simulink model "TP1EJ3_2"  (R2024b)
settings: Solver=VariableStepAuto  StartTime=0.0  StopTime=10.0  FixedStep=0.  RelTol=1e-3
values from neighbouring files (symbols this model uses):
  F = zeros(4,1)    [TP1_Entregable.m]
  Ks = 1.2    [TP1_Entregable.m]
  mur = mus(j)    [TP1_Entregable.m]
  n0 = 0    [TP1_Entregable.m]
  p0 = 0    [TP1_Entregable.m]
  Q = zeros(4,1)    [TP1_Entregable.m]
  s0 = 0    [TP1_Entregable.m]
  s_in = 25    [TP1_Entregable.m]
  v0 = 10    [TP1_Entregable.m]
  x0 = 15    [TP1_Entregable.m]
  xi_in = [0,0; s_in,0; 0,n_in; 0,0]    [TP1_Entregable.m]
undefined symbols (not defined in the file or in its folder): sr
settings Model: Creator=tomii  LastModifiedBy=tomi

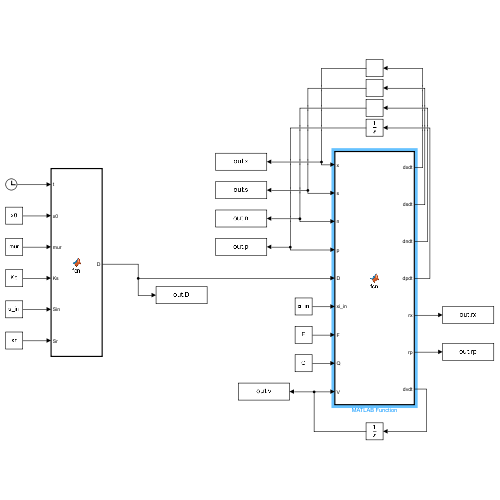
[thumbnail: Simulink's stored preview of the top-level diagram]
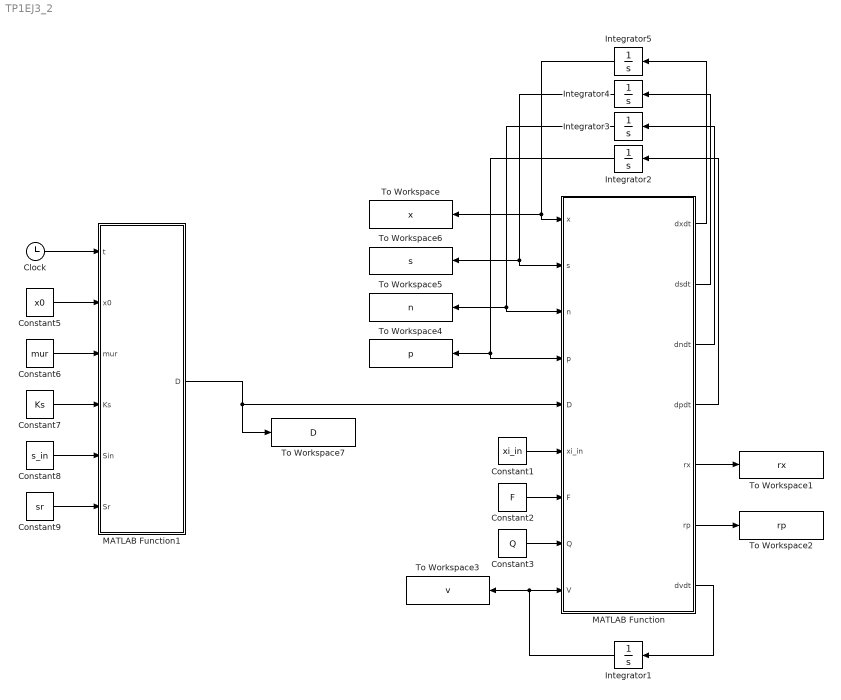
== system TP1EJ3_2 ==
  Clock : Clock
  Constant1 : Constant  Value=xi_in
  Constant2 : Constant  Value=F
  Constant3 : Constant  Value=Q
  Constant5 : Constant  Value=x0
  Constant6 : Constant  Value=mur
  Constant7 : Constant  Value=Ks
  Constant8 : Constant  Value=s_in
  Constant9 : Constant  Value=sr
  Integrator1 : Integrator  InitialCondition=v0
  Integrator2 : Integrator  InitialCondition=p0
  Integrator3 : Integrator  InitialCondition=n0
  Integrator4 : Integrator  InitialCondition=s0
  Integrator5 : Integrator  InitialCondition=x0
  MATLAB Function : MATLAB Function  TreatAsAtomicUnit=on
  MATLAB Function1 : MATLAB Function  TreatAsAtomicUnit=on
  To Workspace : ToWorkspace  VariableName=x  SaveFormat=Timeseries  SampleTime=-1
  To Workspace1 : ToWorkspace  VariableName=rx  SaveFormat=Timeseries  SampleTime=-1
  To Workspace2 : ToWorkspace  VariableName=rp  SaveFormat=Timeseries  SampleTime=-1
  To Workspace3 : ToWorkspace  VariableName=v  SaveFormat=Timeseries  SampleTime=-1
  To Workspace4 : ToWorkspace  VariableName=p  SaveFormat=Timeseries  SampleTime=-1
  To Workspace5 : ToWorkspace  VariableName=n  SaveFormat=Timeseries  SampleTime=-1
  To Workspace6 : ToWorkspace  VariableName=s  SaveFormat=Timeseries  SampleTime=-1
  To Workspace7 : ToWorkspace  VariableName=D  SaveFormat=Timeseries  SampleTime=-1
  wires:
  MATLAB Function1/1(D) -> To Workspace7/1, MATLAB Function/5(D)
  Constant1/1 -> MATLAB Function/6(xi_in)
  Constant2/1 -> MATLAB Function/7(F)
  Constant3/1 -> MATLAB Function/8(Q)
  MATLAB Function/5(rx) -> To Workspace1/1
  MATLAB Function/6(rp) -> To Workspace2/1
  MATLAB Function/7(dvdt) -> Integrator1/1
  Integrator1/1 -> To Workspace3/1, MATLAB Function/9(V)
  MATLAB Function/1(dxdt) -> Integrator5/1
  MATLAB Function/2(dsdt) -> Integrator4/1
  MATLAB Function/3(dndt) -> Integrator3/1
  MATLAB Function/4(dpdt) -> Integrator2/1
  Integrator2/1 -> To Workspace4/1, MATLAB Function/4(p)
  Integrator5/1 -> To Workspace/1, MATLAB Function/1(x)
  Integrator4/1 -> To Workspace6/1, MATLAB Function/2(s)
  Integrator3/1 -> To Workspace5/1, MATLAB Function/3(n)
  Clock/1 -> MATLAB Function1/1(t)
  Constant5/1 -> MATLAB Function1/2(x0)
  Constant8/1 -> MATLAB Function1/5(Sin)
  Constant7/1 -> MATLAB Function1/4(Ks)
  Constant6/1 -> MATLAB Function1/3(mur)
  Constant9/1 -> MATLAB Function1/6(Sr)

== matlab function TP1EJ3_2/MATLAB Function1 ==
  data: t input; D output; x0 input; mur input; Ks input; Sin input; Sr input
function D = fcn(t, x0, mur, Ks, Sin, Sr)
D = (Ks*mur*x0*exp(t*mur))/(Sin-Sr);

== matlab function TP1EJ3_2/MATLAB Function ==
  data: dxdt output; dsdt output; dndt output; dpdt output; x input; s input; n input; p input; D input; xi_in input; F input; Q input; V input; modelParameters parameter; rx output; rp output; dvdt output
function [dxdt, dsdt, dndt, dpdt, rx, rp, dvdt] = fcn(x, s, n, p, D, xi_in, F, Q, V, modelParameters)   
    % Modelo de Monod
    rx_params=modelParameters.rx_params;
    rp_params=modelParameters.rp_params;
    Kipn=modelParameters.Kipn;
    K=modelParameters.K;
    
    rx=HaldaneMonodModel(s, n, rx_params)*n;
    rp=HaldaneMonodModel(s, n, rp_params)*Kipn;

    % states = K * [rx;rp] * x + (xi_in-[x;s;n;p]*[1,1])*[1;1]*D + F - Q;
    states = K * [rx;rp] * x + [0; D*(xi_in(2,1)-s); D*(xi_in(3,2)-n); 0] + F - Q;
    dvdt = D*V;

    dxdt=states(1);
    dsdt=states(2);
    dndt=states(3);
    dpdt=states(4);
end
